simulink model "PV_PerturbAndObserve_MPPT"  (R2022a)
settings: Solver=ode4  StartTime=0.0  StopTime=10.0  FixedStep=5e-6  RelTol=1e-3
libraries: spsSeriesRLCBranchLib x4, spsDiodeLib x1, spsIGBTLib x1, spsPVArrayLib x1, spsPWMGeneratorDCDCLib x1, spsVoltageMeasurementLib x1, spspowerguiLib x1
settings Model: Creator=nikos  LastModifiedBy=nikos

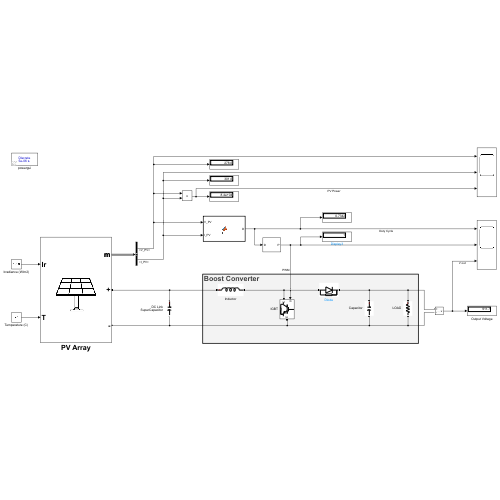
[thumbnail: Simulink's stored preview of the top-level diagram]
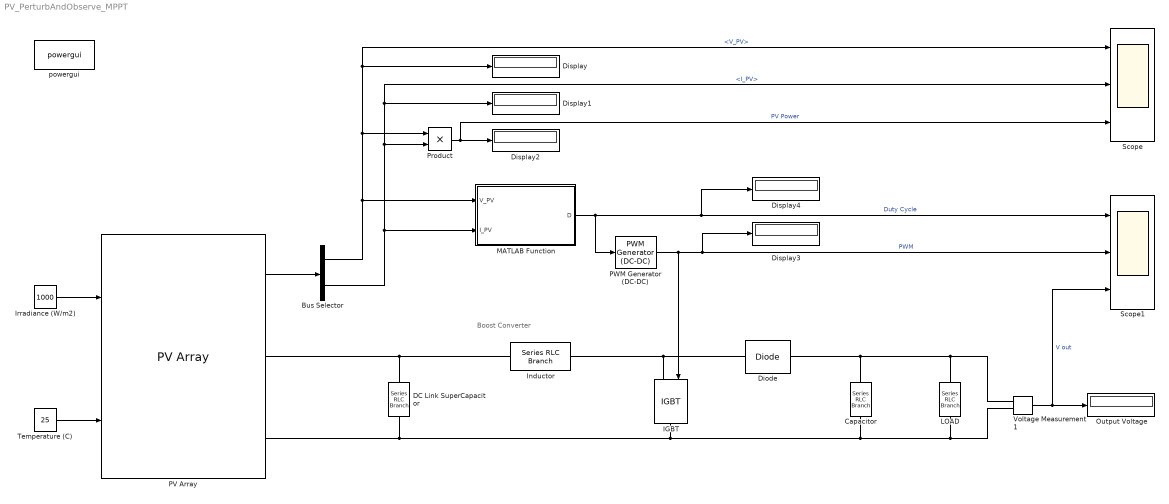
== system PV_PerturbAndObserve_MPPT ==
  note: Boost Converter
  Bus Selector : BusSelector  OutputSignals=V_PV,I_PV
  Capacitor : spsSeriesRLCBranchLib/Series RLC Branch  LConnTagsString=__new0  RConnTagsString=__new0  BranchType=C  Resistance=1  Inductance=1e-3  SetiL0=off  InitialCurrent=0  Capacitance=10e-3  Setx0=off  InitialVoltage=0  Measurements=None
  DC Link SuperCapacitor : spsSeriesRLCBranchLib/Series RLC Branch  LConnTagsString=__new0  RConnTagsString=__new0  BranchType=C  Resistance=1  Inductance=1e-3  SetiL0=off  InitialCurrent=0  Capacitance=100e-6  Setx0=off  InitialVoltage=0  Measurements=None
  Diode : spsDiodeLib/Diode  Ron=0.001  Lon=0  Vf=0.8  IC=0  UseSnubber=0  Rs=500  Cs=250e-9  Measurements=off
  Display{,1..4} (5 alike) : Display
  IGBT : spsIGBTLib/IGBT  Ron=0.001  Lon=0  Vf=1  Tf=1e-6  Tt=2e-6  IC=0  Rs=1e5  Cs=inf  Measurements=off
  Inductor : spsSeriesRLCBranchLib/Series RLC Branch  LConnTagsString=__new0  RConnTagsString=__new0  BranchType=L  Resistance=1  Inductance=1e-3  SetiL0=off  InitialCurrent=0  Capacitance=1e-6  Setx0=off  InitialVoltage=0  Measurements=None
  Irradiance (W/m2) : Constant  Value=1000
  LOAD : spsSeriesRLCBranchLib/Series RLC Branch  LConnTagsString=__new0  RConnTagsString=__new0  BranchType=R  Resistance=10  Inductance=1e-3  SetiL0=off  InitialCurrent=0  Capacitance=1e-6  Setx0=off  InitialVoltage=0  Measurements=None
  MATLAB Function : MATLAB Function  TreatAsAtomicUnit=on
  Output Voltage : Display
  PV Array : spsPVArrayLib/PV Array  Npar=64  Nser=5  PlotType=array @ 1000 W/m2 & specified temperatures  S_vec="[ 1000  500  100 ]"  Temp_C_vec="[ 45 25  ]"  ModuleName=SunPower SPR-315E-WHT-D  PlotWhenSelected=off  Pm=315.072  Ncell=96  Voc=64.6  Isc=6.14  Vm=54.7  Im=5.76  beta_Voc_pc=-0.2727  alpha_Isc_pc=0.061743  beta_Voc=-0.17616  alpha_Isc=0.003791  IL=6.1461  I0=6.5067e-12  nI=0.95071  Rsh=430.0666  Rs=0.43041  RobustModel=off  RobustCellTemperature=313.3991  BAL=on  Tc=1e-6  Tfilter=5e-5
  PWM Generator (DC-DC) : spsPWMGeneratorDCDCLib/PWM Generator (DC-DC)  Fsw=1000  Ts=5e-6
  Product : Product
  Scope : Scope  NumInputPorts=3
  Scope1 : Scope  NumInputPorts=3
  Temperature (C) : Constant  Value=25
  Voltage Measurement1 : spsVoltageMeasurementLib/Voltage Measurement  PhasorSimulation=off  OutputType=Complex  PSBequivalent=0
  powergui : spspowerguiLib/powergui  Priority=1  SimulationMode=Discrete  SampleTime=5e-6  frequency=60  Iterations=50  frequencyindice=0  Pbase=100e6  ErrMax=1e-4  UnitsV=kV  UnitsW=MW  buscounter=0  FunctionMessages=off  echomessages=off  EnableUseOfTLC=off  CurrentSourceSwitches=off  DisableSnubberDevices=off  DisableRonSwitches=off  DisableVfSwitches=off  DisplayEquations=off  AutomaticDiscreteSolvers=off  SolverType=Tustin/Backward Euler (TBE)  Interpol=off  ExternalGateDelay=off  methode=off  Ts=100  x0status=blocks  SPID=on  SwTol=0  HookPort=off  NonlinearTolerance=1e-4  nMaxIteration=100  ContinueOnMaxIteration=off  RestoreLinks=warning  ResistiveCurrentMeasurement=off  Frange=[0:2:500]  Ylog=off  Xlog=on  ShowGrid=off  save=off  variable=ZData  structure=0  ZoomFFT=off  StartTime=0.0  cycles=1  DisplayStyle=1  fundamental=60  FreqAxis=off  MaxFrequency=1000  frequencyindicesteady=1  RmsSteady=1  display=off
  wires:
  Irradiance (W/m2)/1 -> PV Array/1
  Temperature (C)/1 -> PV Array/2
  Product/1 -> Scope/3, Display2/1  "PV Power"
  PWM Generator (DC-DC)/1 -> Display3/1, Scope1/2, IGBT/1  "PWM"
  Voltage Measurement1/1 -> Scope1/3, Output Voltage/1  "V out"
  MATLAB Function/1(D) -> PWM Generator (DC-DC)/1, Display4/1, Scope1/1  "Duty Cycle"
  PV Array/1 -> Bus Selector/1
  Bus Selector/1 -> Product/1, Scope/1, Display/1, MATLAB Function/1(V_PV)  "<V_PV>"
  Bus Selector/2 -> Product/2, Scope/2, Display1/1, MATLAB Function/2(I_PV)  "<I_PV>"
  connections:
  DC Link SuperCapacitor/LConn1 -- Inductor/LConn1 -- PV Array/RConn1
  DC Link SuperCapacitor/RConn1 -- Voltage Measurement1/LConn2 -- LOAD/RConn1 -- Capacitor/RConn1 -- IGBT/RConn1 -- PV Array/RConn2
  IGBT/LConn1 -- Diode/LConn1 -- Inductor/RConn1
  Capacitor/LConn1 -- LOAD/LConn1 -- Voltage Measurement1/LConn1 -- Diode/RConn1

== matlab function PV_PerturbAndObserve_MPPT/MATLAB Function ==
  data: V_PV input; D output; I_PV input
function D = fcn(V_PV, I_PV)

% Initial Duty Cycle with Max and Min Limits 
Dinit = 0.4;
Dmax = 0.9;
Dmin = 0.1;
deltaD = 20e-6;


%Persistent Variables are LOCAL to the Function
persistent Vold Pold Dold;

dataType = "double";

%Initialize these Parameters
if isempty(Vold)
    Vold = 0;
    Pold = 0;
    Dold = Dinit;
end

%P Calculation
P = V_PV * I_PV;
dV = V_PV - Vold;
dP = P - Pold;

%dP<0, dV<0 then Decrease D
%dP<0, dV>0 then Increase D
%dP>0, dV<0 then Increase D
%dP>0, dV>0 then Decrease D
if dP ~= 0 
    if dP < 0
        if dV < 0 
            D = Dold - deltaD;
        else
            D = Dold + deltaD;
        end
        else
        if dV < 0
            D = Dold + deltaD;
        else
            D = Dold - deltaD;
        end
    end
%dP=0 then takes the Old value
    else D = Dold;
end

%if D is more than Max and less than Min then takes the Old Value
if D >= Dmax || D <= Dmin
    D = Dold;
end

%Values Update
Vold = V_PV;
Pold = P;
Dold = D;
